simulink model "SimPrac8"  (R2018a)
settings: Solver=ode45  StartTime=0.0  StopTime=5  RelTol=1e-9
undefined symbols (not defined in the file): K2, Kg, Kr, Ku, Kusil, T1, T1g, T2, T2g, Ung
settings Model: Creator=dirlak  LastModifiedBy=dirlak

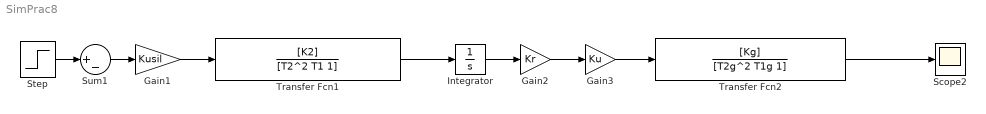
== system SimPrac8 ==
  Gain1 : Gain  Gain=Kusil
  Gain2 : Gain  Gain=Kr
  Gain3 : Gain  Gain=Ku
  Integrator : Integrator
  Scope2 : Scope
  Step : Step  Time=0  After=Ung  SampleTime=0
  Sum1 : Sum  Inputs=|+-
  Transfer Fcn1 : TransferFcn  Numerator=[K2]  Denominator=[T2^2 T1 1]
  Transfer Fcn2 : TransferFcn  Numerator=[Kg]  Denominator=[T2g^2 T1g 1]
  wires:
  Step/1 -> Sum1/1
  Sum1/1 -> Gain1/1
  Gain1/1 -> Transfer Fcn1/1
  Transfer Fcn1/1 -> Integrator/1
  Integrator/1 -> Gain2/1
  Gain2/1 -> Gain3/1
  Gain3/1 -> Transfer Fcn2/1
  Transfer Fcn2/1 -> Scope2/1
